simulink model "HVDCVSCBased"  (R2024b)
settings: Solver=ode45  StartTime=0.0  StopTime=3  FixedStep=Ts_Power  RelTol=1e-3  AbsTol=1e-2
InitFcn:
  | Fnom = 50;        % Hz
  | 
  | Fc = 27*Fnom;   % (Hz)
  | Ts_Power = 1/(Fc*100);
  | Ts_Control = Ts_Power*10;
undefined symbols (not defined in the file or in its folder): D1, Delta, DiscIntNeverNeededParam, magnitude
libraries: spsSecondOrderFilterLib x20, spsSeriesRLCBranchLib x14, spsMeanVariableFrequencyLib x12, spsabctoAlphaBetaZeroLib x8, spsThreePhaseVIMeasurementLib x6, spsAlphaBetaZerotodq0Lib x6, spsCurrentMeasurementLib x4, spsThreePhaseHarmonicFilterLib x4, spsVoltageMeasurementLib x4, spsFirstOrderFilterLib x4, spsGroundLib x3, spsThreePhaseSeriesRLCBranchLib x3
(part 2 of 5)

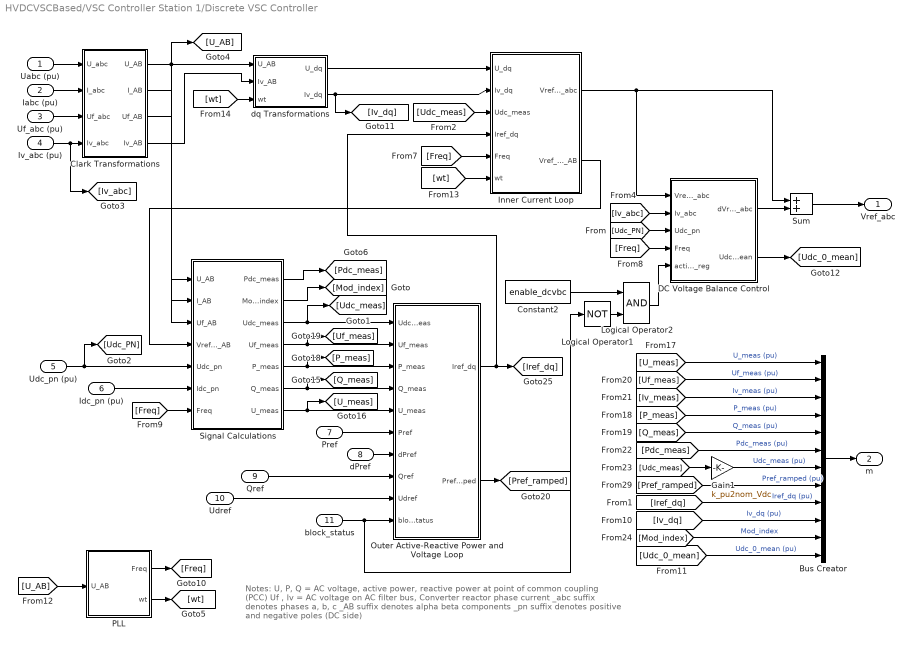
== system HVDCVSCBased/VSC Controller Station 1/Discrete VSC Controller  ==
  note: Notes:
      | U, P, Q = AC voltage, active power, reactive power at point of common coupling (PCC)
      | Uf , Iv  = AC voltage on AC filter bus, Converter reactor phase current
      | _abc suffix denotes phases a, b, c
      | _AB  suffix denotes alpha beta components
      | _pn  suffix denotes positive and negative poles (DC side)
  Uabc (pu) : Inport
  Iabc (pu) : Inport  Port=2
  Uf_abc (pu) : Inport  Port=3
  Iv_abc (pu) : Inport  Port=4
  Udc_pn (pu) : Inport  Port=5
  Idc_pn (pu) : Inport  Port=6
  Pref : Inport  Port=7
  dPref : Inport  Port=8
  Qref : Inport  Port=9
  Udref : Inport  Port=10
  block_status : Inport  Port=11
  Bus Creator : BusCreator  Inputs=12
  Clark Transformations : Subsystem
  Constant2 : Constant  Value=enable_dcvbc
  DC Voltage Balance Control : Subsystem
  Gain1 : Gain  Gain=k_pu2nom_Vdc  SaturateOnIntegerOverflow=on  OutDataTypeStr=Inherit: Same as input  ParamDataTypeStr=Inherit: Same as input
  Inner Current Loop : Subsystem
  Logical Operator1 : Logic  Operator=NOT  Inputs=1  AllPortsSameDT=off
  Logical Operator2 : Logic  AllPortsSameDT=off
  Outer Active-Reactive Power and Voltage Loop : Subsystem
  PLL : Subsystem  mask(Discrete 3-phase PLL){Fmin=f_min_pll, Par_Init=[0   Fnom], ParK=[Kp_pll  Ki_pll], Ts=Ts_Control}
      mask prompts: Fmin "Minimum frequency (Hz):"; Par_Init "Initial inputs:[ Phase(degrees)   Frequency(Hz) ]"; ParK "Regulator gains [ Kp  Ki ]"; Ts "Sample time:"
      mask help:
      | This Phase Locked Loop (PLL) system can be used  to synchronize on a set of variable frequency, three-phase sinusoidal signals.
      |
      | Input 1: Vector containing the normalized
      |              three-phase signals [Va Vb Vc]
      | Output 1:  Measured frequency (Hz) = w/(2pi)
      | Output 2:  Ramp w.t   varying between  0 and 2*pi,
      | synchronized on zero crossings of the fundamental (positive-sequence) of phase A.
      | Output 3: Vector [sin(wt) cos(wt)]
      mask init:
      | Kp=ParK(1);
      | Ki=ParK(2);
      | Phase_Init=Par_Init(1);
      | Finit=Par_Init(2);
  Signal Calculations : Subsystem
  Sum : Sum  SaturateOnIntegerOverflow=on
  dq Transformations : Subsystem
  Vref_abc : Outport  VectorParamsAs1DForOutWhenUnconnected=off
  m : Outport  Port=2  VectorParamsAs1DForOutWhenUnconnected=off
  wires:
  PLL/2(wt) -> [wt]
  PLL/1(Freq) -> [Freq]
  Outer Active-Reactive Power and Voltage Loop/1(Iref_dq) -> Inner Current Loop/4(Iref_dq), [Iref_dq]
  dq Transformations/2(Iv_dq) -> [Iv_dq], Inner Current Loop/2(Iv_dq)
  Inner Current Loop/1(Vref_lim_abc) -> Sum/1, DC Voltage Balance Control/1(Vref_lim_abc)
  dq Transformations/1(U_dq) -> Inner Current Loop/1(U_dq)
  Signal Calculations/3(Udc_meas) -> Outer Active-Reactive Power and Voltage Loop/1(Udc_meas), [Udc_meas]
  Signal Calculations/4(Uf_meas) -> Outer Active-Reactive Power and Voltage Loop/2(Uf_meas), [Uf_meas]
  Signal Calculations/6(Q_meas) -> Outer Active-Reactive Power and Voltage Loop/4(Q_meas), [Q_meas]
  Signal Calculations/5(P_meas) -> Outer Active-Reactive Power and Voltage Loop/3(P_meas), [P_meas]
  Clark Transformations/1(U_AB) -> dq Transformations/1(U_AB), Signal Calculations/1(U_AB), [U_AB]
  Signal Calculations/1(Pdc_meas) -> [Pdc_meas]
  Constant2/1 -> Logical Operator2/1
  Pref/1 -> Outer Active-Reactive Power and Voltage Loop/6(Pref)
  dPref/1 -> Outer Active-Reactive Power and Voltage Loop/7(dPref)
  Qref/1 -> Outer Active-Reactive Power and Voltage Loop/8(Qref)
  Logical Operator2/1 -> DC Voltage Balance Control/5(activate_reg)
  [Udc_PN] -> DC Voltage Balance Control/3(Udc_pn)
  Udc_pn (pu)/1 -> Signal Calculations/5(Udc_pn), [Udc_PN]
  [Iv_abc] -> DC Voltage Balance Control/2(Iv_abc)
  Idc_pn (pu)/1 -> Signal Calculations/6(Idc_pn)
  [Freq] -> Inner Current Loop/5(Freq)
  [Freq] -> DC Voltage Balance Control/4(Freq)
  [Freq] -> Signal Calculations/7(Freq)
  Clark Transformations/2(I_AB) -> Signal Calculations/2(I_AB)
  [U_AB] -> PLL/1(U_AB)
  [wt] -> Inner Current Loop/6(wt)
  [wt] -> dq Transformations/3(wt)
  block_status/1 -> Outer Active-Reactive Power and Voltage Loop/10(block_status), Logical Operator1/1
  Signal Calculations/7(U_meas) -> Outer Active-Reactive Power and Voltage Loop/5(U_meas), [U_meas]
  Sum/1 -> Vref_abc/1
  Logical Operator1/1 -> Logical Operator2/2
  [Udc_meas] -> Inner Current Loop/3(Udc_meas)
  Signal Calculations/2(Mod_index) -> [Mod_index]
  DC Voltage Balance Control/1(dVref_abc) -> Sum/2
  Clark Transformations/4(Iv_AB) -> dq Transformations/2(Iv_AB)
  Clark Transformations/3(Uf_AB) -> Signal Calculations/3(Uf_AB)
  Udref/1 -> Outer Active-Reactive Power and Voltage Loop/9(Udref)
  Bus Creator/1 -> m/1
  [U_meas] -> Bus Creator/1  "U_meas (pu)"
  [P_meas] -> Bus Creator/4  "P_meas (pu)"
  [Uf_meas] -> Bus Creator/2  "Uf_meas (pu)"
  [Iv_meas] -> Bus Creator/3  "Iv_meas (pu)"
  Outer Active-Reactive Power and Voltage Loop/2(Pref_ramped) -> [Pref_ramped]
  [Pref_ramped] -> Bus Creator/8  "Pref_ramped (pu)"
  Inner Current Loop/2(Vref_lim_AB) -> Signal Calculations/4(Vref_lim_AB)
  [Iv_dq] -> Bus Creator/10  "Iv_dq (pu)"
  DC Voltage Balance Control/2(Udc_0_mean) -> [Udc_0_mean]
  [Udc_0_mean] -> Bus Creator/12  "Udc_0_mean (pu)"
  Uabc (pu)/1 -> Clark Transformations/1("U_abc ")
  Iabc (pu)/1 -> Clark Transformations/2("I_abc ")
  Uf_abc (pu)/1 -> Clark Transformations/3("Uf_abc ")
  Iv_abc (pu)/1 -> Clark Transformations/4("Iv_abc "), [Iv_abc]
  [Q_meas] -> Bus Creator/5  "Q_meas (pu)"
  [Pdc_meas] -> Bus Creator/6  "Pdc_meas (pu)"
  [Iref_dq] -> Bus Creator/9  "Iref_dq (pu)"
  [Mod_index] -> Bus Creator/11  "Mod_index"
  Gain1/1 -> Bus Creator/7  "Udc_meas (pu)"
  [Udc_meas] -> Gain1/1

== system HVDCVSCBased/VSC Controller Station 2/Anti-aliasing Filters ==
  note: Filtering
  note: Low-pass filter
  "Uabc " : Inport  PortDimensions=3
  "Iabc " : Inport  Port=2  PortDimensions=3
  "Uf_abc  " : Inport  Port=3  PortDimensions=3
  "Iv_abc " : Inport  Port=4  PortDimensions=3
  "Udc_pn  " : Inport  Port=5
  "Idc_pn " : Inport  Port=6
  Second-Order Filter{,1..5} (6 alike) : spsSecondOrderFilterLib/Second-Order Filter  FilterType=Lowpass  Fo=f0_aa  Zeta=zeta  Ts=Ts_Control  Initialize=off  Vac_Init="[0,  0,  60]"  Vdc_Init=0  PlotResponse=off  FreqRange=[0, 500, 1]
      settings: AttributesFormatString=f0=%<Fo>
  Uabc : Outport  VectorParamsAs1DForOutWhenUnconnected=off
  Iabc : Outport  Port=2  VectorParamsAs1DForOutWhenUnconnected=off
  Uf_abc : Outport  Port=3  VectorParamsAs1DForOutWhenUnconnected=off
  " Iv_abc" : Outport  Port=4  VectorParamsAs1DForOutWhenUnconnected=off
  "Udc_pn " : Outport  Port=5  VectorParamsAs1DForOutWhenUnconnected=off
  " Idc_pn" : Outport  Port=6  VectorParamsAs1DForOutWhenUnconnected=off
  wires:
  "Iv_abc "/1 -> Second-Order Filter/1
  Second-Order Filter/1 -> " Iv_abc"/1
  "Uf_abc  "/1 -> Second-Order Filter1/1
  Second-Order Filter1/1 -> Uf_abc/1
  "Uabc "/1 -> Second-Order Filter2/1
  Second-Order Filter2/1 -> Uabc/1
  "Udc_pn  "/1 -> Second-Order Filter3/1
  Second-Order Filter3/1 -> "Udc_pn "/1
  "Idc_pn "/1 -> Second-Order Filter4/1
  Second-Order Filter4/1 -> " Idc_pn"/1
  "Iabc "/1 -> Second-Order Filter5/1
  Second-Order Filter5/1 -> Iabc/1

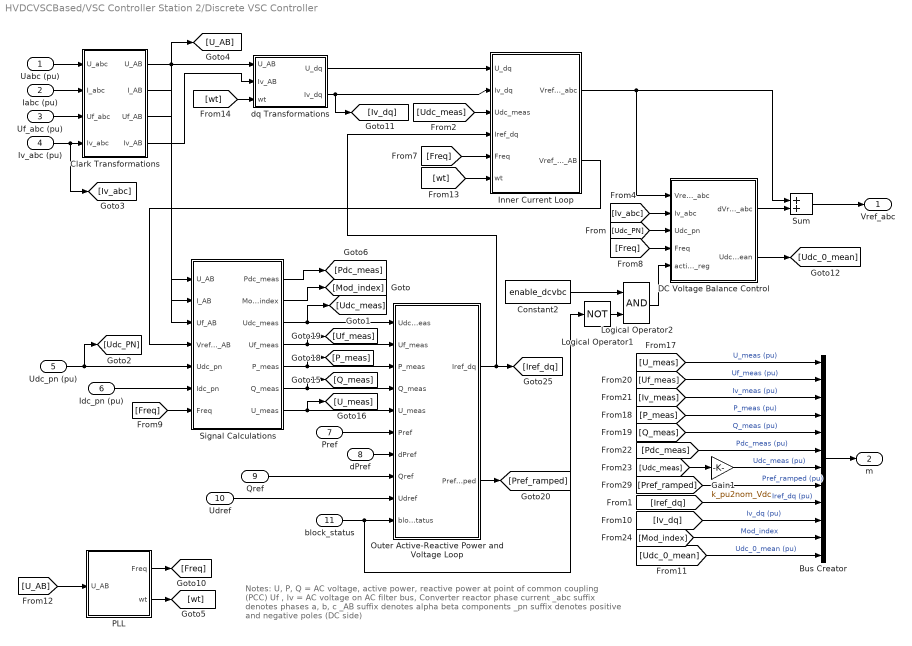
== system HVDCVSCBased/VSC Controller Station 2/Discrete VSC Controller  ==
  note: Notes:
      | U, P, Q = AC voltage, active power, reactive power at point of common coupling (PCC)
      | Uf , Iv  = AC voltage on AC filter bus, Converter reactor phase current
      | _abc suffix denotes phases a, b, c
      | _AB  suffix denotes alpha beta components
      | _pn  suffix denotes positive and negative poles (DC side)
  Uabc (pu) : Inport
  Iabc (pu) : Inport  Port=2
  Uf_abc (pu) : Inport  Port=3
  Iv_abc (pu) : Inport  Port=4
  Udc_pn (pu) : Inport  Port=5
  Idc_pn (pu) : Inport  Port=6
  Pref : Inport  Port=7
  dPref : Inport  Port=8
  Qref : Inport  Port=9
  Udref : Inport  Port=10
  block_status : Inport  Port=11
  Bus Creator : BusCreator  Inputs=12
  Clark Transformations : Subsystem
  Constant2 : Constant  Value=enable_dcvbc
  DC Voltage Balance Control : Subsystem
  Gain1 : Gain  Gain=k_pu2nom_Vdc  SaturateOnIntegerOverflow=on  OutDataTypeStr=Inherit: Same as input  ParamDataTypeStr=Inherit: Same as input
  Inner Current Loop : Subsystem
  Logical Operator1 : Logic  Operator=NOT  Inputs=1  AllPortsSameDT=off
  Logical Operator2 : Logic  AllPortsSameDT=off
  Outer Active-Reactive Power and Voltage Loop : Subsystem
  PLL : Subsystem  mask(Discrete 3-phase PLL){Fmin=f_min_pll, Par_Init=[0   Fnom], ParK=[Kp_pll  Ki_pll], Ts=Ts_Control}
      mask prompts: Fmin "Minimum frequency (Hz):"; Par_Init "Initial inputs:[ Phase(degrees)   Frequency(Hz) ]"; ParK "Regulator gains [ Kp  Ki ]"; Ts "Sample time:"
      mask help:
      | This Phase Locked Loop (PLL) system can be used  to synchronize on a set of variable frequency, three-phase sinusoidal signals.
      |
      | Input 1: Vector containing the normalized
      |              three-phase signals [Va Vb Vc]
      | Output 1:  Measured frequency (Hz) = w/(2pi)
      | Output 2:  Ramp w.t   varying between  0 and 2*pi,
      | synchronized on zero crossings of the fundamental (positive-sequence) of phase A.
      | Output 3: Vector [sin(wt) cos(wt)]
      mask init:
      | Kp=ParK(1);
      | Ki=ParK(2);
      | Phase_Init=Par_Init(1);
      | Finit=Par_Init(2);
  Signal Calculations : Subsystem
  Sum : Sum  SaturateOnIntegerOverflow=on
  dq Transformations : Subsystem
  Vref_abc : Outport  VectorParamsAs1DForOutWhenUnconnected=off
  m : Outport  Port=2  VectorParamsAs1DForOutWhenUnconnected=off
  wires:
  PLL/2(wt) -> [wt]
  PLL/1(Freq) -> [Freq]
  Outer Active-Reactive Power and Voltage Loop/1(Iref_dq) -> Inner Current Loop/4(Iref_dq), [Iref_dq]
  dq Transformations/2(Iv_dq) -> [Iv_dq], Inner Current Loop/2(Iv_dq)
  Inner Current Loop/1(Vref_lim_abc) -> Sum/1, DC Voltage Balance Control/1(Vref_lim_abc)
  dq Transformations/1(U_dq) -> Inner Current Loop/1(U_dq)
  Signal Calculations/3(Udc_meas) -> Outer Active-Reactive Power and Voltage Loop/1(Udc_meas), [Udc_meas]
  Signal Calculations/4(Uf_meas) -> Outer Active-Reactive Power and Voltage Loop/2(Uf_meas), [Uf_meas]
  Signal Calculations/6(Q_meas) -> Outer Active-Reactive Power and Voltage Loop/4(Q_meas), [Q_meas]
  Signal Calculations/5(P_meas) -> Outer Active-Reactive Power and Voltage Loop/3(P_meas), [P_meas]
  Clark Transformations/1(U_AB) -> dq Transformations/1(U_AB), Signal Calculations/1(U_AB), [U_AB]
  Signal Calculations/1(Pdc_meas) -> [Pdc_meas]
  Constant2/1 -> Logical Operator2/1
  Pref/1 -> Outer Active-Reactive Power and Voltage Loop/6(Pref)
  dPref/1 -> Outer Active-Reactive Power and Voltage Loop/7(dPref)
  Qref/1 -> Outer Active-Reactive Power and Voltage Loop/8(Qref)
  Logical Operator2/1 -> DC Voltage Balance Control/5(activate_reg)
  [Udc_PN] -> DC Voltage Balance Control/3(Udc_pn)
  Udc_pn (pu)/1 -> Signal Calculations/5(Udc_pn), [Udc_PN]
  [Iv_abc] -> DC Voltage Balance Control/2(Iv_abc)
  Idc_pn (pu)/1 -> Signal Calculations/6(Idc_pn)
  [Freq] -> Inner Current Loop/5(Freq)
  [Freq] -> DC Voltage Balance Control/4(Freq)
  [Freq] -> Signal Calculations/7(Freq)
  Clark Transformations/2(I_AB) -> Signal Calculations/2(I_AB)
  [U_AB] -> PLL/1(U_AB)
  [wt] -> Inner Current Loop/6(wt)
  [wt] -> dq Transformations/3(wt)
  block_status/1 -> Outer Active-Reactive Power and Voltage Loop/10(block_status), Logical Operator1/1
  Signal Calculations/7(U_meas) -> Outer Active-Reactive Power and Voltage Loop/5(U_meas), [U_meas]
  Sum/1 -> Vref_abc/1
  Logical Operator1/1 -> Logical Operator2/2
  [Udc_meas] -> Inner Current Loop/3(Udc_meas)
  Signal Calculations/2(Mod_index) -> [Mod_index]
  DC Voltage Balance Control/1(dVref_abc) -> Sum/2
  Clark Transformations/4(Iv_AB) -> dq Transformations/2(Iv_AB)
  Clark Transformations/3(Uf_AB) -> Signal Calculations/3(Uf_AB)
  Udref/1 -> Outer Active-Reactive Power and Voltage Loop/9(Udref)
  Bus Creator/1 -> m/1
  [U_meas] -> Bus Creator/1  "U_meas (pu)"
  [P_meas] -> Bus Creator/4  "P_meas (pu)"
  [Uf_meas] -> Bus Creator/2  "Uf_meas (pu)"
  [Iv_meas] -> Bus Creator/3  "Iv_meas (pu)"
  Outer Active-Reactive Power and Voltage Loop/2(Pref_ramped) -> [Pref_ramped]
  [Pref_ramped] -> Bus Creator/8  "Pref_ramped (pu)"
  Inner Current Loop/2(Vref_lim_AB) -> Signal Calculations/4(Vref_lim_AB)
  [Iv_dq] -> Bus Creator/10  "Iv_dq (pu)"
  DC Voltage Balance Control/2(Udc_0_mean) -> [Udc_0_mean]
  [Udc_0_mean] -> Bus Creator/12  "Udc_0_mean (pu)"
  Uabc (pu)/1 -> Clark Transformations/1("U_abc ")
  Iabc (pu)/1 -> Clark Transformations/2("I_abc ")
  Uf_abc (pu)/1 -> Clark Transformations/3("Uf_abc ")
  Iv_abc (pu)/1 -> Clark Transformations/4("Iv_abc "), [Iv_abc]
  [Q_meas] -> Bus Creator/5  "Q_meas (pu)"
  [Pdc_meas] -> Bus Creator/6  "Pdc_meas (pu)"
  [Iref_dq] -> Bus Creator/9  "Iref_dq (pu)"
  [Mod_index] -> Bus Creator/11  "Mod_index"
  Gain1/1 -> Bus Creator/7  "Udc_meas (pu)"
  [Udc_meas] -> Gain1/1

== system HVDCVSCBased/VSC Controller Station 1/Discrete VSC Controller /Clark Transformations ==
  note: 0: Y-Y
      | 1: Y-D1
      | 2: Y-D11
  note: Clark's Transformations
  "U_abc " : Inport
  "I_abc " : Inport  Port=2
  "Uf_abc " : Inport  Port=3
  "Iv_abc " : Inport  Port=4
  CLARK  with Rotating reference : Subsystem
  CLARK  with Rotating reference1 : Subsystem
  Constant2 : Constant  Value=Tr_connection
  Selector{,1..3} (4 alike) : Selector  InputPortWidth=3  IndexOptions=Index vector (dialog)  Indices=[1 2]  OutputSizes=1
  abc to Alpha-Beta-Zero : spsabctoAlphaBetaZeroLib/abc to Alpha-Beta-Zero
  abc to Alpha-Beta-Zero1 : spsabctoAlphaBetaZeroLib/abc to Alpha-Beta-Zero
  U_AB : Outport  VectorParamsAs1DForOutWhenUnconnected=off
  I_AB : Outport  Port=2  VectorParamsAs1DForOutWhenUnconnected=off
  Uf_AB : Outport  Port=3  VectorParamsAs1DForOutWhenUnconnected=off
  Iv_AB : Outport  Port=4  VectorParamsAs1DForOutWhenUnconnected=off
  wires:
  Constant2/1 -> CLARK  with Rotating reference/2(Type), CLARK  with Rotating reference1/2(Type)
  "U_abc "/1 -> CLARK  with Rotating reference/1(abc)
  "I_abc "/1 -> CLARK  with Rotating reference1/1(abc)
  "Uf_abc "/1 -> abc to Alpha-Beta-Zero/1
  "Iv_abc "/1 -> abc to Alpha-Beta-Zero1/1
  CLARK  with Rotating reference/1(AB0) -> Selector/1
  abc to Alpha-Beta-Zero/1 -> Selector2/1
  abc to Alpha-Beta-Zero1/1 -> Selector3/1
  CLARK  with Rotating reference1/1(AB0) -> Selector1/1
  Selector/1 -> U_AB/1
  Selector1/1 -> I_AB/1
  Selector2/1 -> Uf_AB/1
  Selector3/1 -> Iv_AB/1

== system HVDCVSCBased/VSC Controller Station 1/Discrete VSC Controller /DC Voltage Balance Control ==
  note: DC Voltage Balance Control
  note: pu AC ==> pu DC
  Vref_lim_abc : Inport
  Iv_abc : Inport  Port=2
  Udc_pn : Inport  Port=3
  Freq : Inport  Port=4
  activate_reg : Inport  Port=5
  Constant8 : Constant  Value=0
  First-Order Filter : spsFirstOrderFilterLib/First-Order Filter  FilterType=Lowpass  Tc=1/(2*pi*f0_dcvbc)  Ts=Ts_Control  Initialize=off  Vac_Init=[0, 0, 60]  Vdc_Init=0  PlotResponse=off  FreqRange="[0,  200,  1]"
      settings: AttributesFormatString=Tc:%<Tc>
  Gain4 : Gain  Gain=k_pu2nom_Vdc  SaturateOnIntegerOverflow=on  OutDataTypeStr=Inherit: Same as input  ParamDataTypeStr=Inherit: Same as input
  Mean (Variable Frequency) : spsMeanVariableFrequencyLib/Mean (Variable Frequency)  Finit=Fnom  Fmin=f_min_pll  Vinit=0  Ts=Ts_Control
  Regulator : Subsystem  TreatAsAtomicUnit=on
  Sum : Sum  Inputs=1  SaturateOnIntegerOverflow=on
  Switch2 : Switch  Criteria=u2 > Threshold  InputSameDT=off
  dVref_abc : Outport  VectorParamsAs1DForOutWhenUnconnected=off
  Udc_0_mean : Outport  Port=2  VectorParamsAs1DForOutWhenUnconnected=off
  wires:
  First-Order Filter/1 -> Mean (Variable Frequency)/2
  Sum/1 -> First-Order Filter/1
  Freq/1 -> Mean (Variable Frequency)/1
  Vref_lim_abc/1 -> Regulator/1(V_ref_lim_abc)
  Iv_abc/1 -> Regulator/2(Iv_abc)
  Udc_pn/1 -> Sum/1
  Mean (Variable Frequency)/1 -> Gain4/1
  Gain4/1 -> Regulator/3(Udc_0_mean), Udc_0_mean/1
  Regulator/1(dV_ref_abc_dcvbc) -> Switch2/1
  Switch2/1 -> dVref_abc/1
  Constant8/1 -> Switch2/3
  activate_reg/1 -> Regulator/Enable, Switch2/2

== system HVDCVSCBased/VSC Controller Station 1/Discrete VSC Controller /Inner Current Loop ==
  note: Inner Current Loop
  U_dq : Inport
  Iv_dq : Inport  Port=2
  Udc_meas : Inport  Port=3
  Iref_dq : Inport  Port=4
  Freq : Inport  Port=5
  wt : Inport  Port=6
  AC_Current_Control : Subsystem
  Alpha-Beta-Zero to abc : spsAlphaBetaZerotoabcLib/Alpha-Beta-Zero to abc
  Constant1 : Constant  Value=0
  Max=10 Min=0 : Saturate  UpperLimit=10  LowerLimit=0
  Mean (Variable Frequency IC = 1.0 ) : spsMeanVariableFrequencyLib/Mean (Variable Frequency)  Finit=Fnom  Fmin=f_min_pll  Vinit=1.0  Ts=Ts_Control
  Mux1 : Mux  Inputs=[2 1]
  Reference_Voltage_Conditioning : Subsystem
  Reference_Voltage_Limitation : Subsystem
  Selector : Selector  InputPortWidth=3  IndexOptions=Index vector (dialog)  Indices=[ 1 2]  OutputSizes=1
  dq0 to Alpha-Beta-Zero : spsdq0toAlphaBetaZeroLib/dq0 to Alpha-Beta-Zero  Alignment=90 degrees behind phase A axis
  Vref_lim_abc : Outport  VectorParamsAs1DForOutWhenUnconnected=off
  Vref_lim_AB : Outport  Port=2  VectorParamsAs1DForOutWhenUnconnected=off
  wires:
  Udc_meas/1 -> Mean (Variable Frequency IC = 1.0 )/2
  Selector/1 -> Vref_lim_AB/1
  Reference_Voltage_Limitation/1(Vref_lim_dq) -> Mux1/1
  Alpha-Beta-Zero to abc/1 -> Vref_lim_abc/1
  Mux1/1 -> dq0 to Alpha-Beta-Zero/1
  Constant1/1 -> Mux1/2
  wt/1 -> dq0 to Alpha-Beta-Zero/2
  dq0 to Alpha-Beta-Zero/1 -> Selector/1, Alpha-Beta-Zero to abc/1
  Mean (Variable Frequency IC = 1.0 )/1 -> Max=10 Min=0/1
  Freq/1 -> Mean (Variable Frequency IC = 1.0 )/1, AC_Current_Control/4(Freq)
  Iref_dq/1 -> AC_Current_Control/2(Iref_dq)
  U_dq/1 -> AC_Current_Control/3(U_dq)
  Reference_Voltage_Conditioning/1(Vref_dq) -> Reference_Voltage_Limitation/1(Vref_dq)
  AC_Current_Control/1(Vref_dq_tmp) -> Reference_Voltage_Conditioning/1(Vref_dq_tmp)
  Max=10 Min=0/1 -> Reference_Voltage_Conditioning/2(Udc_meas_mean)
  Iv_dq/1 -> AC_Current_Control/1(Iv_dq)

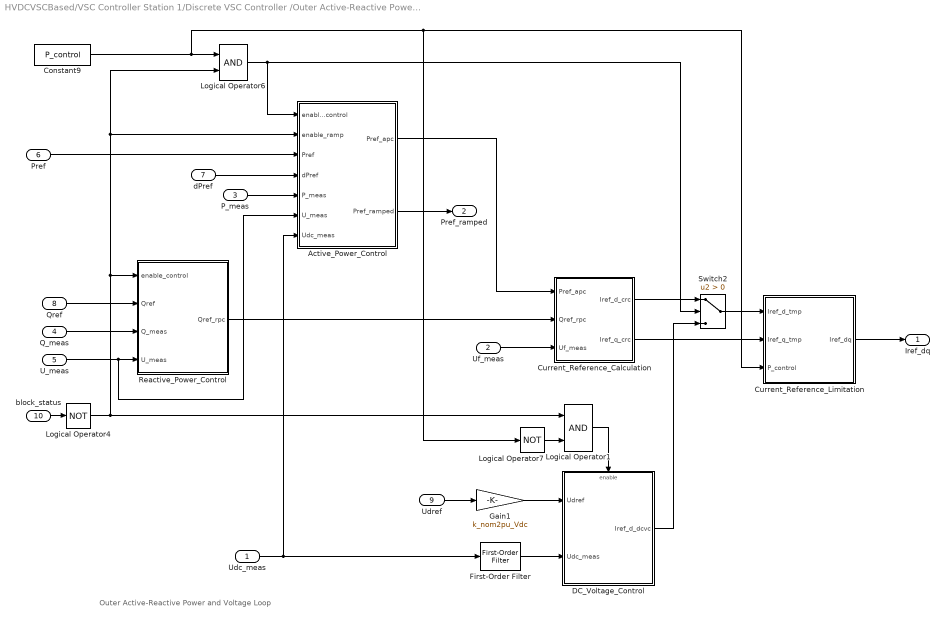
== system HVDCVSCBased/VSC Controller Station 1/Discrete VSC Controller /Outer Active-Reactive Power and Voltage Loop ==
  note: Outer Active-Reactive Power and Voltage Loop
  Udc_meas : Inport
  Uf_meas : Inport  Port=2
  P_meas : Inport  Port=3
  Q_meas : Inport  Port=4
  U_meas : Inport  Port=5
  Pref : Inport  Port=6
  dPref : Inport  Port=7
  Qref : Inport  Port=8
  Udref : Inport  Port=9
  block_status : Inport  Port=10
  Active_Power_Control : Subsystem
  Constant9 : Constant  Value=P_control
  Current_Reference_Calculation : Subsystem
  Current_Reference_Limitation : Subsystem
  DC_Voltage_Control : Subsystem
  First-Order Filter : spsFirstOrderFilterLib/First-Order Filter  FilterType=Lowpass  Tc=1/(2*pi*f0_Udc)  Ts=Ts_Control  Initialize=on  Vac_Init=[0, 0, 60]  Vdc_Init=k_nom2pu_Vdc  PlotResponse=off  FreqRange="[0,  200,  1]"
      settings: AttributesFormatString=Tc:%<Tc>\nIC:%<Vdc_Init>
  Gain1 : Gain  Gain=k_nom2pu_Vdc  SaturateOnIntegerOverflow=on  OutDataTypeStr=Inherit: Same as input  ParamDataTypeStr=Inherit: Same as input
      settings: AttributesFormatString=Gain:%<Gain>
  Logical Operator1 : Logic  AllPortsSameDT=off
  Logical Operator4 : Logic  Operator=NOT  AllPortsSameDT=off
  Logical Operator6 : Logic  AllPortsSameDT=off
  Logical Operator7 : Logic  Operator=NOT  AllPortsSameDT=off
  Reactive_Power_Control : Subsystem
  Switch2 : Switch  Criteria=u2 > Threshold  InputSameDT=off
  Iref_dq : Outport  VectorParamsAs1DForOutWhenUnconnected=off
  Pref_ramped : Outport  Port=2  VectorParamsAs1DForOutWhenUnconnected=off
  wires:
  First-Order Filter/1 -> DC_Voltage_Control/2(Udc_meas)
  Udref/1 -> Gain1/1
  Gain1/1 -> DC_Voltage_Control/1(Udref)
  Logical Operator1/1 -> DC_Voltage_Control/Enable
  Current_Reference_Limitation/1(Iref_dq) -> Iref_dq/1
  Switch2/1 -> Current_Reference_Limitation/1(Iref_d_tmp)
  Logical Operator4/1 -> Logical Operator1/1, Logical Operator6/2, Active_Power_Control/2(enable_ramp), Reactive_Power_Control/1(enable_control)
  Current_Reference_Calculation/1(Iref_d_crc) -> Switch2/1
  Q_meas/1 -> Reactive_Power_Control/3(Q_meas)
  P_meas/1 -> Active_Power_Control/5(P_meas)
  DC_Voltage_Control/1(Iref_d_dcvc) -> Switch2/3
  Udc_meas/1 -> Active_Power_Control/7(Udc_meas), First-Order Filter/1
  block_status/1 -> Logical Operator4/1
  Constant9/1 -> Logical Operator6/1, Current_Reference_Limitation/3(P_control), Logical Operator7/1
  Logical Operator6/1 -> Switch2/2, Active_Power_Control/1(enable_control)
  U_meas/1 -> Reactive_Power_Control/4(U_meas), Active_Power_Control/6(U_meas)
  Current_Reference_Calculation/2(Iref_q_crc) -> Current_Reference_Limitation/2(Iref_q_tmp)
  dPref/1 -> Active_Power_Control/4(dPref)
  Active_Power_Control/1(Pref_apc) -> Current_Reference_Calculation/1(Pref_apc)
  Reactive_Power_Control/1(Qref_rpc) -> Current_Reference_Calculation/2(Qref_rpc)
  Pref/1 -> Active_Power_Control/3(Pref)
  Uf_meas/1 -> Current_Reference_Calculation/3(Uf_meas)
  Qref/1 -> Reactive_Power_Control/2(Qref)
  Logical Operator7/1 -> Logical Operator1/2
  Active_Power_Control/2(Pref_ramped) -> Pref_ramped/1

== system HVDCVSCBased/VSC Controller Station 1/Discrete VSC Controller /PLL ==
  note: Discrete 3-phase PLL (Variation)
  U_AB : Inport
  Alpha-Beta-Zero to dq0 : spsAlphaBetaZerotodq0Lib/Alpha-Beta-Zero to dq0  Alignment=90 degrees behind phase A axis
  Constant1 : Constant  Value=0
  Constant4 : Constant  Value=2*pi
  Discrete PI Controller : Subsystem  DialogController=POWERSYS.PowerSysDialog  mask(Discrete PI Controller){Kp=Kp, Ki=Ki, Par_Limits=2*pi*Finit*[1.25 0.75], Init=2*pi*Finit, Ts=Ts}
      mask prompts: Kp "Proportional gain (Kp):"; Ki "Integral gain (Ki):"; Par_Limits "Output limits: [ Upper   Lower ]"; Init "Output initial value:"; Ts "Sample time:"
      mask help: This block implements a discrete PI controller.
      mask init:
      | UpperLimit=Par_Limits(1);
      | LowerLimit=Par_Limits(2);
      | power_initmask();
      mask Help: This block is part of a subset of blocks in the Extras library that does not have documentation associated with it, other than the block mask description.
      mask Display: disp('PI');
  Discrete Rate Limiter : Subsystem  DialogController=POWERSYS.PowerSysDialog  mask(Discrete Rate Limiter){R=12, F=-12, Vinit=Finit, Ts=Ts}
      mask prompts: R "Rising slew rate:"; F "Falling slew rate:"; Vinit "Initial input:"; Ts "Sample time:"
      mask help: DISCRETE BLOCK : Limit rising and falling rates of signal
      mask init:
      | UpperLimit=R*Ts;
      | LowerLimit=F*Ts;
      | power_initmask();
      mask Help: This block is part of a subset of blocks in the Extras library that does not have documentation associated with it, other than the block mask description.
      mask Display: disp('Discrete\nRate\nLimiter')
  Discrete-Time Integrator : DiscreteIntegrator  InitialCondition=Phase_Init*pi/180  SampleTime=Ts  ICPrevOutput=DiscIntNeverNeededParam  ICPrevScaledInput=DiscIntNeverNeededParam
  Gain10 : Gain  Gain=1/2/pi  SaturateOnIntegerOverflow=on  OutDataTypeStr=Inherit: Same as input  ParamDataTypeStr=Inherit: Same as input
  Math Function : Math  Operator=mod  SignedPower=on
  Mean (Variable Frequency) : spsMeanVariableFrequencyLib/Mean (Variable Frequency)  Finit=Finit  Fmin=Fmin  Vinit=0  Ts=Ts
  Mux1 : Mux  Inputs=[2 1]
  Second-Order Filter : spsSecondOrderFilterLib/Second-Order Filter  FilterType=Lowpass  Fo=25  Zeta=0.707  Ts=Ts  Initialize=on  Vac_Init=[0 0 Finit]  Vdc_Init=Finit  PlotResponse=off  FreqRange=[0, 500, 1]
  Selector : Selector  InputPortWidth=3  IndexOptions=Index vector (dialog)  Indices=2  OutputSizes=1
  Unit Delay : UnitDelay  InitialCondition=Finit  SampleTime=Ts  HasFrameUpgradeWarning=on
  Freq : Outport  VectorParamsAs1DForOutWhenUnconnected=off
  wt : Outport  Port=2  VectorParamsAs1DForOutWhenUnconnected=off
  wires:
  Constant1/1 -> Mux1/2
  Mux1/1 -> Alpha-Beta-Zero to dq0/1
  U_AB/1 -> Mux1/1
  Mean (Variable Frequency)/1 -> Discrete PI Controller/1(Error)
  Alpha-Beta-Zero to dq0/1 -> Selector/1
  Constant4/1 -> Math Function/2
  Discrete-Time Integrator/1 -> Math Function/1
  Math Function/1 -> wt/1, Alpha-Beta-Zero to dq0/2
  Discrete PI Controller/1(Out) -> Discrete-Time Integrator/1, Gain10/1  "W"
  Gain10/1 -> Discrete Rate Limiter/1(In)
  Discrete Rate Limiter/1(Out) -> Second-Order Filter/1
  Unit Delay/1 -> Freq/1, Mean (Variable Frequency)/1
  Second-Order Filter/1 -> Unit Delay/1
  Selector/1 -> Mean (Variable Frequency)/2  "Vq"

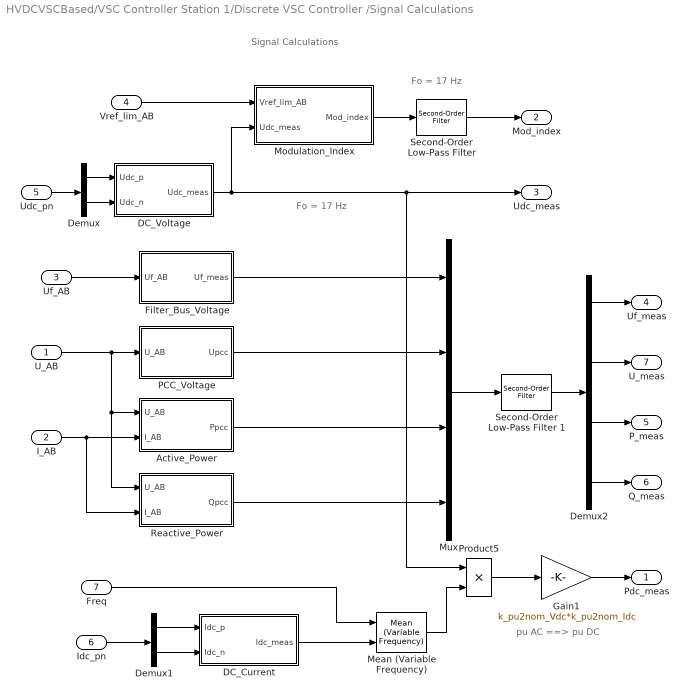
== system HVDCVSCBased/VSC Controller Station 1/Discrete VSC Controller /Signal Calculations ==
  note: Fo = 17 Hz
  note: Fo = 17 Hz
  note: Signal Calculations
  note: pu AC ==> pu DC
  U_AB : Inport
  I_AB : Inport  Port=2
  Uf_AB : Inport  Port=3
  Vref_lim_AB : Inport  Port=4
  Udc_pn : Inport  Port=5
  Idc_pn : Inport  Port=6
  Freq : Inport  Port=7
  Active_Power : Subsystem
  DC_Current : Subsystem
  DC_Voltage : Subsystem
  Demux : Demux  Outputs=2
      settings: DisplayOption=none
  Demux1 : Demux  Outputs=2
      settings: DisplayOption=none
  Demux2 : Demux
  Filter_Bus_Voltage : Subsystem
  Gain1 : Gain  Gain=k_pu2nom_Vdc*k_pu2nom_Idc  SaturateOnIntegerOverflow=on  OutDataTypeStr=Inherit: Same as input  ParamDataTypeStr=Inherit: Same as input
  "Mean (Variable Frequency) " : spsMeanVariableFrequencyLib/Mean (Variable Frequency)  Finit=Fnom  Fmin=f_min_pll  Vinit=0  Ts=Ts_Control
  Modulation_Index : Subsystem
  Mux : Mux
  PCC_Voltage : Subsystem
  Product5 : Product  SaturateOnIntegerOverflow=on  OutDataTypeStr=Inherit: Same as first input
  Reactive_Power : Subsystem
  "Second-Order Low-Pass Filter " : spsSecondOrderFilterLib/Second-Order Filter  FilterType=Lowpass  Fo=f0_sc  Zeta=zeta_sc  Ts=Ts_Control  Initialize=off  Vac_Init="[0,  0,  60]"  Vdc_Init=0  PlotResponse=off  FreqRange=[0, 500, 1]
      settings: AttributesFormatString=f0=%<Fo>
  Second-Order Low-Pass Filter 1 : spsSecondOrderFilterLib/Second-Order Filter  FilterType=Lowpass  Fo=f0_sc  Zeta=zeta_sc  Ts=Ts_Control  Initialize=off  Vac_Init="[0,  0,  60]"  Vdc_Init=0  PlotResponse=off  FreqRange=[0, 500, 1]
      settings: AttributesFormatString=f0=%<Fo>
  Pdc_meas : Outport  VectorParamsAs1DForOutWhenUnconnected=off
  Mod_index : Outport  Port=2  VectorParamsAs1DForOutWhenUnconnected=off
  Udc_meas : Outport  Port=3  VectorParamsAs1DForOutWhenUnconnected=off
  Uf_meas : Outport  Port=4  VectorParamsAs1DForOutWhenUnconnected=off
  P_meas : Outport  Port=5  VectorParamsAs1DForOutWhenUnconnected=off
  Q_meas : Outport  Port=6  VectorParamsAs1DForOutWhenUnconnected=off
  U_meas : Outport  Port=7  VectorParamsAs1DForOutWhenUnconnected=off
  wires:
  Demux2/4 -> Q_meas/1
  Demux2/3 -> P_meas/1
  Demux2/2 -> U_meas/1
  Demux2/1 -> Uf_meas/1
  Reactive_Power/1(Qpcc) -> Mux/4
  Active_Power/1(Ppcc) -> Mux/3
  PCC_Voltage/1(Upcc) -> Mux/2
  Filter_Bus_Voltage/1(Uf_meas) -> Mux/1
  "Second-Order Low-Pass Filter "/1 -> Mod_index/1
  Modulation_Index/1(Mod_index) -> "Second-Order Low-Pass Filter "/1
  Second-Order Low-Pass Filter 1/1 -> Demux2/1
  Mux/1 -> Second-Order Low-Pass Filter 1/1
  Gain1/1 -> Pdc_meas/1
  Freq/1 -> "Mean (Variable Frequency) "/1
  Product5/1 -> Gain1/1
  "Mean (Variable Frequency) "/1 -> Product5/2
  Demux/2 -> DC_Voltage/2(Udc_n)
  Uf_AB/1 -> Filter_Bus_Voltage/1(Uf_AB)
  U_AB/1 -> PCC_Voltage/1(U_AB), Active_Power/1(U_AB), Reactive_Power/1(U_AB)
  I_AB/1 -> Active_Power/2(I_AB), Reactive_Power/2(I_AB)
  DC_Voltage/1(Udc_meas) -> Product5/1, Udc_meas/1, Modulation_Index/2(Udc_meas)
  DC_Current/1(Idc_meas) -> "Mean (Variable Frequency) "/2
  Udc_pn/1 -> Demux/1
  Demux/1 -> DC_Voltage/1(Udc_p)
  Demux1/1 -> DC_Current/1(Idc_p)
  Demux1/2 -> DC_Current/2(Idc_n)
  Idc_pn/1 -> Demux1/1
  Vref_lim_AB/1 -> Modulation_Index/1(Vref_lim_AB)

== system HVDCVSCBased/VSC Controller Station 1/Discrete VSC Controller /dq Transformations ==
  note: dq Transformations
  U_AB : Inport
  Iv_AB : Inport  Port=2
  wt : Inport  Port=3
  Alpha-Beta-Zero to dq0 : spsAlphaBetaZerotodq0Lib/Alpha-Beta-Zero to dq0  Alignment=90 degrees behind phase A axis
  "Alpha-Beta-Zero to dq0 " : spsAlphaBetaZerotodq0Lib/Alpha-Beta-Zero to dq0  Alignment=90 degrees behind phase A axis
  Constant1 : Constant  Value=0
  Mux1 : Mux  Inputs=[2 1]
  Mux4 : Mux  Inputs=[2 1]
  Selector : Selector  InputPortWidth=3  IndexOptions=Index vector (dialog)  Indices=[1 2]  OutputSizes=1
  Selector3 : Selector  InputPortWidth=3  IndexOptions=Index vector (dialog)  Indices=[1 2]  OutputSizes=1
  U_dq : Outport  VectorParamsAs1DForOutWhenUnconnected=off
  Iv_dq : Outport  Port=2  VectorParamsAs1DForOutWhenUnconnected=off
  wires:
  wt/1 -> Alpha-Beta-Zero to dq0/2, "Alpha-Beta-Zero to dq0 "/2
  Constant1/1 -> Mux4/2, Mux1/2
  Mux4/1 -> "Alpha-Beta-Zero to dq0 "/1
  Iv_AB/1 -> Mux4/1
  Mux1/1 -> Alpha-Beta-Zero to dq0/1
  U_AB/1 -> Mux1/1
  "Alpha-Beta-Zero to dq0 "/1 -> Selector3/1
  Alpha-Beta-Zero to dq0/1 -> Selector/1
  Selector/1 -> U_dq/1
  Selector3/1 -> Iv_dq/1

== system HVDCVSCBased/VSC Controller Station 2/Discrete VSC Controller /Clark Transformations ==
  note: 0: Y-Y
      | 1: Y-D1
      | 2: Y-D11
  note: Clark's Transformations
  "U_abc " : Inport
  "I_abc " : Inport  Port=2
  "Uf_abc " : Inport  Port=3
  "Iv_abc " : Inport  Port=4
  CLARK  with Rotating reference : Subsystem
  CLARK  with Rotating reference1 : Subsystem
  Constant2 : Constant  Value=Tr_connection
  Selector{,1..3} (4 alike) : Selector  InputPortWidth=3  IndexOptions=Index vector (dialog)  Indices=[1 2]  OutputSizes=1
  abc to Alpha-Beta-Zero : spsabctoAlphaBetaZeroLib/abc to Alpha-Beta-Zero
  abc to Alpha-Beta-Zero1 : spsabctoAlphaBetaZeroLib/abc to Alpha-Beta-Zero
  U_AB : Outport  VectorParamsAs1DForOutWhenUnconnected=off
  I_AB : Outport  Port=2  VectorParamsAs1DForOutWhenUnconnected=off
  Uf_AB : Outport  Port=3  VectorParamsAs1DForOutWhenUnconnected=off
  Iv_AB : Outport  Port=4  VectorParamsAs1DForOutWhenUnconnected=off
  wires:
  Constant2/1 -> CLARK  with Rotating reference/2(Type), CLARK  with Rotating reference1/2(Type)
  "U_abc "/1 -> CLARK  with Rotating reference/1(abc)
  "I_abc "/1 -> CLARK  with Rotating reference1/1(abc)
  "Uf_abc "/1 -> abc to Alpha-Beta-Zero/1
  "Iv_abc "/1 -> abc to Alpha-Beta-Zero1/1
  CLARK  with Rotating reference/1(AB0) -> Selector/1
  abc to Alpha-Beta-Zero/1 -> Selector2/1
  abc to Alpha-Beta-Zero1/1 -> Selector3/1
  CLARK  with Rotating reference1/1(AB0) -> Selector1/1
  Selector/1 -> U_AB/1
  Selector1/1 -> I_AB/1
  Selector2/1 -> Uf_AB/1
  Selector3/1 -> Iv_AB/1

== system HVDCVSCBased/VSC Controller Station 2/Discrete VSC Controller /DC Voltage Balance Control ==
  note: DC Voltage Balance Control
  note: pu AC ==> pu DC
  Vref_lim_abc : Inport
  Iv_abc : Inport  Port=2
  Udc_pn : Inport  Port=3
  Freq : Inport  Port=4
  activate_reg : Inport  Port=5
  Constant8 : Constant  Value=0
  First-Order Filter : spsFirstOrderFilterLib/First-Order Filter  FilterType=Lowpass  Tc=1/(2*pi*f0_dcvbc)  Ts=Ts_Control  Initialize=off  Vac_Init=[0, 0, 60]  Vdc_Init=0  PlotResponse=off  FreqRange="[0,  200,  1]"
      settings: AttributesFormatString=Tc:%<Tc>
  Gain4 : Gain  Gain=k_pu2nom_Vdc  SaturateOnIntegerOverflow=on  OutDataTypeStr=Inherit: Same as input  ParamDataTypeStr=Inherit: Same as input
  Mean (Variable Frequency) : spsMeanVariableFrequencyLib/Mean (Variable Frequency)  Finit=Fnom  Fmin=f_min_pll  Vinit=0  Ts=Ts_Control
  Regulator : Subsystem  TreatAsAtomicUnit=on
  Sum : Sum  Inputs=1  SaturateOnIntegerOverflow=on
  Switch2 : Switch  Criteria=u2 > Threshold  InputSameDT=off
  dVref_abc : Outport  VectorParamsAs1DForOutWhenUnconnected=off
  Udc_0_mean : Outport  Port=2  VectorParamsAs1DForOutWhenUnconnected=off
  wires:
  First-Order Filter/1 -> Mean (Variable Frequency)/2
  Sum/1 -> First-Order Filter/1
  Freq/1 -> Mean (Variable Frequency)/1
  Vref_lim_abc/1 -> Regulator/1(V_ref_lim_abc)
  Iv_abc/1 -> Regulator/2(Iv_abc)
  Udc_pn/1 -> Sum/1
  Mean (Variable Frequency)/1 -> Gain4/1
  Gain4/1 -> Regulator/3(Udc_0_mean), Udc_0_mean/1
  Regulator/1(dV_ref_abc_dcvbc) -> Switch2/1
  Switch2/1 -> dVref_abc/1
  Constant8/1 -> Switch2/3
  activate_reg/1 -> Regulator/Enable, Switch2/2

== system HVDCVSCBased/VSC Controller Station 2/Discrete VSC Controller /Inner Current Loop ==
  note: Inner Current Loop
  U_dq : Inport
  Iv_dq : Inport  Port=2
  Udc_meas : Inport  Port=3
  Iref_dq : Inport  Port=4
  Freq : Inport  Port=5
  wt : Inport  Port=6
  AC_Current_Control : Subsystem
  Alpha-Beta-Zero to abc : spsAlphaBetaZerotoabcLib/Alpha-Beta-Zero to abc
  Constant1 : Constant  Value=0
  Max=10 Min=0 : Saturate  UpperLimit=10  LowerLimit=0
  Mean (Variable Frequency IC = 1.0 ) : spsMeanVariableFrequencyLib/Mean (Variable Frequency)  Finit=Fnom  Fmin=f_min_pll  Vinit=1.0  Ts=Ts_Control
  Mux1 : Mux  Inputs=[2 1]
  Reference_Voltage_Conditioning : Subsystem
  Reference_Voltage_Limitation : Subsystem
  Selector : Selector  InputPortWidth=3  IndexOptions=Index vector (dialog)  Indices=[ 1 2]  OutputSizes=1
  dq0 to Alpha-Beta-Zero : spsdq0toAlphaBetaZeroLib/dq0 to Alpha-Beta-Zero  Alignment=90 degrees behind phase A axis
  Vref_lim_abc : Outport  VectorParamsAs1DForOutWhenUnconnected=off
  Vref_lim_AB : Outport  Port=2  VectorParamsAs1DForOutWhenUnconnected=off
  wires:
  Udc_meas/1 -> Mean (Variable Frequency IC = 1.0 )/2
  Selector/1 -> Vref_lim_AB/1
  Reference_Voltage_Limitation/1(Vref_lim_dq) -> Mux1/1
  Alpha-Beta-Zero to abc/1 -> Vref_lim_abc/1
  Mux1/1 -> dq0 to Alpha-Beta-Zero/1
  Constant1/1 -> Mux1/2
  wt/1 -> dq0 to Alpha-Beta-Zero/2
  dq0 to Alpha-Beta-Zero/1 -> Selector/1, Alpha-Beta-Zero to abc/1
  Mean (Variable Frequency IC = 1.0 )/1 -> Max=10 Min=0/1
  Freq/1 -> Mean (Variable Frequency IC = 1.0 )/1, AC_Current_Control/4(Freq)
  Iref_dq/1 -> AC_Current_Control/2(Iref_dq)
  U_dq/1 -> AC_Current_Control/3(U_dq)
  Reference_Voltage_Conditioning/1(Vref_dq) -> Reference_Voltage_Limitation/1(Vref_dq)
  AC_Current_Control/1(Vref_dq_tmp) -> Reference_Voltage_Conditioning/1(Vref_dq_tmp)
  Max=10 Min=0/1 -> Reference_Voltage_Conditioning/2(Udc_meas_mean)
  Iv_dq/1 -> AC_Current_Control/1(Iv_dq)

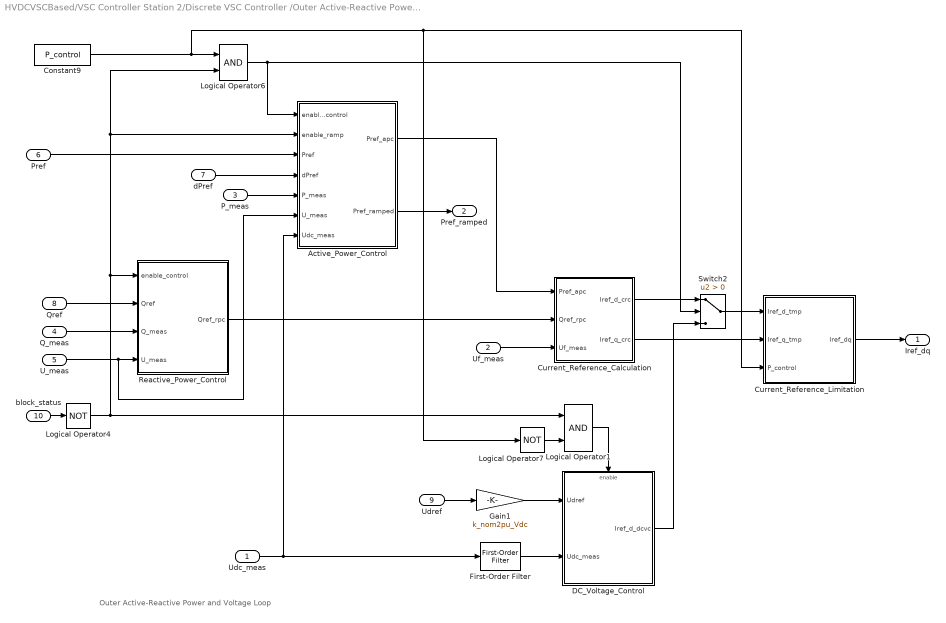
== system HVDCVSCBased/VSC Controller Station 2/Discrete VSC Controller /Outer Active-Reactive Power and Voltage Loop ==
  note: Outer Active-Reactive Power and Voltage Loop
  Udc_meas : Inport
  Uf_meas : Inport  Port=2
  P_meas : Inport  Port=3
  Q_meas : Inport  Port=4
  U_meas : Inport  Port=5
  Pref : Inport  Port=6
  dPref : Inport  Port=7
  Qref : Inport  Port=8
  Udref : Inport  Port=9
  block_status : Inport  Port=10
  Active_Power_Control : Subsystem
  Constant9 : Constant  Value=P_control
  Current_Reference_Calculation : Subsystem
  Current_Reference_Limitation : Subsystem
  DC_Voltage_Control : Subsystem
  First-Order Filter : spsFirstOrderFilterLib/First-Order Filter  FilterType=Lowpass  Tc=1/(2*pi*f0_Udc)  Ts=Ts_Control  Initialize=on  Vac_Init=[0, 0, 60]  Vdc_Init=k_nom2pu_Vdc  PlotResponse=off  FreqRange="[0,  200,  1]"
      settings: AttributesFormatString=Tc:%<Tc>\nIC:%<Vdc_Init>
  Gain1 : Gain  Gain=k_nom2pu_Vdc  SaturateOnIntegerOverflow=on  OutDataTypeStr=Inherit: Same as input  ParamDataTypeStr=Inherit: Same as input
      settings: AttributesFormatString=Gain:%<Gain>
  Logical Operator1 : Logic  AllPortsSameDT=off
  Logical Operator4 : Logic  Operator=NOT  AllPortsSameDT=off
  Logical Operator6 : Logic  AllPortsSameDT=off
  Logical Operator7 : Logic  Operator=NOT  AllPortsSameDT=off
  Reactive_Power_Control : Subsystem
  Switch2 : Switch  Criteria=u2 > Threshold  InputSameDT=off
  Iref_dq : Outport  VectorParamsAs1DForOutWhenUnconnected=off
  Pref_ramped : Outport  Port=2  VectorParamsAs1DForOutWhenUnconnected=off
  wires:
  First-Order Filter/1 -> DC_Voltage_Control/2(Udc_meas)
  Udref/1 -> Gain1/1
  Gain1/1 -> DC_Voltage_Control/1(Udref)
  Logical Operator1/1 -> DC_Voltage_Control/Enable
  Current_Reference_Limitation/1(Iref_dq) -> Iref_dq/1
  Switch2/1 -> Current_Reference_Limitation/1(Iref_d_tmp)
  Logical Operator4/1 -> Logical Operator1/1, Logical Operator6/2, Active_Power_Control/2(enable_ramp), Reactive_Power_Control/1(enable_control)
  Current_Reference_Calculation/1(Iref_d_crc) -> Switch2/1
  Q_meas/1 -> Reactive_Power_Control/3(Q_meas)
  P_meas/1 -> Active_Power_Control/5(P_meas)
  DC_Voltage_Control/1(Iref_d_dcvc) -> Switch2/3
  Udc_meas/1 -> Active_Power_Control/7(Udc_meas), First-Order Filter/1
  block_status/1 -> Logical Operator4/1
  Constant9/1 -> Logical Operator6/1, Current_Reference_Limitation/3(P_control), Logical Operator7/1
  Logical Operator6/1 -> Switch2/2, Active_Power_Control/1(enable_control)
  U_meas/1 -> Reactive_Power_Control/4(U_meas), Active_Power_Control/6(U_meas)
  Current_Reference_Calculation/2(Iref_q_crc) -> Current_Reference_Limitation/2(Iref_q_tmp)
  dPref/1 -> Active_Power_Control/4(dPref)
  Active_Power_Control/1(Pref_apc) -> Current_Reference_Calculation/1(Pref_apc)
  Reactive_Power_Control/1(Qref_rpc) -> Current_Reference_Calculation/2(Qref_rpc)
  Pref/1 -> Active_Power_Control/3(Pref)
  Uf_meas/1 -> Current_Reference_Calculation/3(Uf_meas)
  Qref/1 -> Reactive_Power_Control/2(Qref)
  Logical Operator7/1 -> Logical Operator1/2
  Active_Power_Control/2(Pref_ramped) -> Pref_ramped/1

== system HVDCVSCBased/VSC Controller Station 2/Discrete VSC Controller /PLL ==
  note: Discrete 3-phase PLL (Variation)
  U_AB : Inport
  Alpha-Beta-Zero to dq0 : spsAlphaBetaZerotodq0Lib/Alpha-Beta-Zero to dq0  Alignment=90 degrees behind phase A axis
  Constant1 : Constant  Value=0
  Constant4 : Constant  Value=2*pi
  Discrete PI Controller : Subsystem  DialogController=POWERSYS.PowerSysDialog  mask(Discrete PI Controller){Kp=Kp, Ki=Ki, Par_Limits=2*pi*Finit*[1.25 0.75], Init=2*pi*Finit, Ts=Ts}
      mask prompts: Kp "Proportional gain (Kp):"; Ki "Integral gain (Ki):"; Par_Limits "Output limits: [ Upper   Lower ]"; Init "Output initial value:"; Ts "Sample time:"
      mask help: This block implements a discrete PI controller.
      mask init:
      | UpperLimit=Par_Limits(1);
      | LowerLimit=Par_Limits(2);
      | power_initmask();
      mask Help: This block is part of a subset of blocks in the Extras library that does not have documentation associated with it, other than the block mask description.
      mask Display: disp('PI');
  Discrete Rate Limiter : Subsystem  DialogController=POWERSYS.PowerSysDialog  mask(Discrete Rate Limiter){R=12, F=-12, Vinit=Finit, Ts=Ts}
      mask prompts: R "Rising slew rate:"; F "Falling slew rate:"; Vinit "Initial input:"; Ts "Sample time:"
      mask help: DISCRETE BLOCK : Limit rising and falling rates of signal
      mask init:
      | UpperLimit=R*Ts;
      | LowerLimit=F*Ts;
      | power_initmask();
      mask Help: This block is part of a subset of blocks in the Extras library that does not have documentation associated with it, other than the block mask description.
      mask Display: disp('Discrete\nRate\nLimiter')
  Discrete-Time Integrator : DiscreteIntegrator  InitialCondition=Phase_Init*pi/180  SampleTime=Ts  ICPrevOutput=DiscIntNeverNeededParam  ICPrevScaledInput=DiscIntNeverNeededParam
  Gain10 : Gain  Gain=1/2/pi  SaturateOnIntegerOverflow=on  OutDataTypeStr=Inherit: Same as input  ParamDataTypeStr=Inherit: Same as input
  Math Function : Math  Operator=mod  SignedPower=on
  Mean (Variable Frequency) : spsMeanVariableFrequencyLib/Mean (Variable Frequency)  Finit=Finit  Fmin=Fmin  Vinit=0  Ts=Ts
  Mux1 : Mux  Inputs=[2 1]
  Second-Order Filter : spsSecondOrderFilterLib/Second-Order Filter  FilterType=Lowpass  Fo=25  Zeta=0.707  Ts=Ts  Initialize=on  Vac_Init=[0 0 Finit]  Vdc_Init=Finit  PlotResponse=off  FreqRange=[0, 500, 1]
  Selector : Selector  InputPortWidth=3  IndexOptions=Index vector (dialog)  Indices=2  OutputSizes=1
  Unit Delay : UnitDelay  InitialCondition=Finit  SampleTime=Ts  HasFrameUpgradeWarning=on
  Freq : Outport  VectorParamsAs1DForOutWhenUnconnected=off
  wt : Outport  Port=2  VectorParamsAs1DForOutWhenUnconnected=off
  wires:
  Constant1/1 -> Mux1/2
  Mux1/1 -> Alpha-Beta-Zero to dq0/1
  U_AB/1 -> Mux1/1
  Mean (Variable Frequency)/1 -> Discrete PI Controller/1(Error)
  Alpha-Beta-Zero to dq0/1 -> Selector/1
  Constant4/1 -> Math Function/2
  Discrete-Time Integrator/1 -> Math Function/1
  Math Function/1 -> wt/1, Alpha-Beta-Zero to dq0/2
  Discrete PI Controller/1(Out) -> Discrete-Time Integrator/1, Gain10/1  "W"
  Gain10/1 -> Discrete Rate Limiter/1(In)
  Discrete Rate Limiter/1(Out) -> Second-Order Filter/1
  Unit Delay/1 -> Freq/1, Mean (Variable Frequency)/1
  Second-Order Filter/1 -> Unit Delay/1
  Selector/1 -> Mean (Variable Frequency)/2  "Vq"

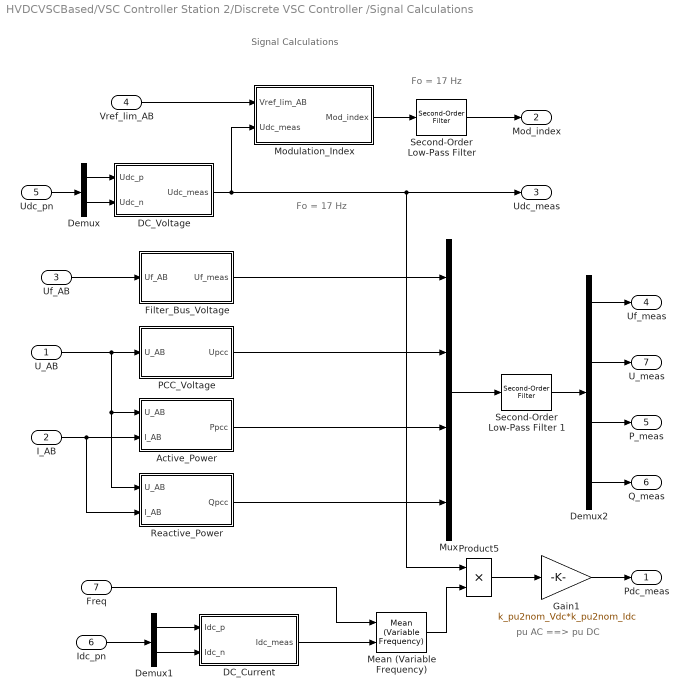
== system HVDCVSCBased/VSC Controller Station 2/Discrete VSC Controller /Signal Calculations ==
  note: Fo = 17 Hz
  note: Fo = 17 Hz
  note: Signal Calculations
  note: pu AC ==> pu DC
  U_AB : Inport
  I_AB : Inport  Port=2
  Uf_AB : Inport  Port=3
  Vref_lim_AB : Inport  Port=4
  Udc_pn : Inport  Port=5
  Idc_pn : Inport  Port=6
  Freq : Inport  Port=7
  Active_Power : Subsystem
  DC_Current : Subsystem
  DC_Voltage : Subsystem
  Demux : Demux  Outputs=2
      settings: DisplayOption=none
  Demux1 : Demux  Outputs=2
      settings: DisplayOption=none
  Demux2 : Demux
  Filter_Bus_Voltage : Subsystem
  Gain1 : Gain  Gain=k_pu2nom_Vdc*k_pu2nom_Idc  SaturateOnIntegerOverflow=on  OutDataTypeStr=Inherit: Same as input  ParamDataTypeStr=Inherit: Same as input
  "Mean (Variable Frequency) " : spsMeanVariableFrequencyLib/Mean (Variable Frequency)  Finit=Fnom  Fmin=f_min_pll  Vinit=0  Ts=Ts_Control
  Modulation_Index : Subsystem
  Mux : Mux
  PCC_Voltage : Subsystem
  Product5 : Product  SaturateOnIntegerOverflow=on  OutDataTypeStr=Inherit: Same as first input
  Reactive_Power : Subsystem
  "Second-Order Low-Pass Filter " : spsSecondOrderFilterLib/Second-Order Filter  FilterType=Lowpass  Fo=f0_sc  Zeta=zeta_sc  Ts=Ts_Control  Initialize=off  Vac_Init="[0,  0,  60]"  Vdc_Init=0  PlotResponse=off  FreqRange=[0, 500, 1]
      settings: AttributesFormatString=f0=%<Fo>
  Second-Order Low-Pass Filter 1 : spsSecondOrderFilterLib/Second-Order Filter  FilterType=Lowpass  Fo=f0_sc  Zeta=zeta_sc  Ts=Ts_Control  Initialize=off  Vac_Init="[0,  0,  60]"  Vdc_Init=0  PlotResponse=off  FreqRange=[0, 500, 1]
      settings: AttributesFormatString=f0=%<Fo>
  Pdc_meas : Outport  VectorParamsAs1DForOutWhenUnconnected=off
  Mod_index : Outport  Port=2  VectorParamsAs1DForOutWhenUnconnected=off
  Udc_meas : Outport  Port=3  VectorParamsAs1DForOutWhenUnconnected=off
  Uf_meas : Outport  Port=4  VectorParamsAs1DForOutWhenUnconnected=off
  P_meas : Outport  Port=5  VectorParamsAs1DForOutWhenUnconnected=off
  Q_meas : Outport  Port=6  VectorParamsAs1DForOutWhenUnconnected=off
  U_meas : Outport  Port=7  VectorParamsAs1DForOutWhenUnconnected=off
  wires:
  Demux2/4 -> Q_meas/1
  Demux2/3 -> P_meas/1
  Demux2/2 -> U_meas/1
  Demux2/1 -> Uf_meas/1
  Reactive_Power/1(Qpcc) -> Mux/4
  Active_Power/1(Ppcc) -> Mux/3
  PCC_Voltage/1(Upcc) -> Mux/2
  Filter_Bus_Voltage/1(Uf_meas) -> Mux/1
  "Second-Order Low-Pass Filter "/1 -> Mod_index/1
  Modulation_Index/1(Mod_index) -> "Second-Order Low-Pass Filter "/1
  Second-Order Low-Pass Filter 1/1 -> Demux2/1
  Mux/1 -> Second-Order Low-Pass Filter 1/1
  Gain1/1 -> Pdc_meas/1
  Freq/1 -> "Mean (Variable Frequency) "/1
  Product5/1 -> Gain1/1
  "Mean (Variable Frequency) "/1 -> Product5/2
  Demux/2 -> DC_Voltage/2(Udc_n)
  Uf_AB/1 -> Filter_Bus_Voltage/1(Uf_AB)
  U_AB/1 -> PCC_Voltage/1(U_AB), Active_Power/1(U_AB), Reactive_Power/1(U_AB)
  I_AB/1 -> Active_Power/2(I_AB), Reactive_Power/2(I_AB)
  DC_Voltage/1(Udc_meas) -> Product5/1, Udc_meas/1, Modulation_Index/2(Udc_meas)
  DC_Current/1(Idc_meas) -> "Mean (Variable Frequency) "/2
  Udc_pn/1 -> Demux/1
  Demux/1 -> DC_Voltage/1(Udc_p)
  Demux1/1 -> DC_Current/1(Idc_p)
  Demux1/2 -> DC_Current/2(Idc_n)
  Idc_pn/1 -> Demux1/1
  Vref_lim_AB/1 -> Modulation_Index/1(Vref_lim_AB)

== system HVDCVSCBased/VSC Controller Station 2/Discrete VSC Controller /dq Transformations ==
  note: dq Transformations
  U_AB : Inport
  Iv_AB : Inport  Port=2
  wt : Inport  Port=3
  Alpha-Beta-Zero to dq0 : spsAlphaBetaZerotodq0Lib/Alpha-Beta-Zero to dq0  Alignment=90 degrees behind phase A axis
  "Alpha-Beta-Zero to dq0 " : spsAlphaBetaZerotodq0Lib/Alpha-Beta-Zero to dq0  Alignment=90 degrees behind phase A axis
  Constant1 : Constant  Value=0
  Mux1 : Mux  Inputs=[2 1]
  Mux4 : Mux  Inputs=[2 1]
  Selector : Selector  InputPortWidth=3  IndexOptions=Index vector (dialog)  Indices=[1 2]  OutputSizes=1
  Selector3 : Selector  InputPortWidth=3  IndexOptions=Index vector (dialog)  Indices=[1 2]  OutputSizes=1
  U_dq : Outport  VectorParamsAs1DForOutWhenUnconnected=off
  Iv_dq : Outport  Port=2  VectorParamsAs1DForOutWhenUnconnected=off
  wires:
  wt/1 -> Alpha-Beta-Zero to dq0/2, "Alpha-Beta-Zero to dq0 "/2
  Constant1/1 -> Mux4/2, Mux1/2
  Mux4/1 -> "Alpha-Beta-Zero to dq0 "/1
  Iv_AB/1 -> Mux4/1
  Mux1/1 -> Alpha-Beta-Zero to dq0/1
  U_AB/1 -> Mux1/1
  "Alpha-Beta-Zero to dq0 "/1 -> Selector3/1
  Alpha-Beta-Zero to dq0/1 -> Selector/1
  Selector/1 -> U_dq/1
  Selector3/1 -> Iv_dq/1

== system HVDCVSCBased/VSC Controller Station 1/Discrete VSC Controller /Clark Transformations/CLARK  with Rotating reference ==
  note: Rotation of pi/6
  note: Rotation of - pi/6
  note: Reference rotation:
      | Type [0,1,2]          Rotation (rad)
      | 0                            0
      | 1                            - pi/6
      | 2                              pi/6
  note: CLARK transformations
  abc : Inport
  Type : Inport  Port=2
  CLARK : Subsystem  TreatAsAtomicUnit=on
  CLARK_lag : Subsystem  TreatAsAtomicUnit=on
  CLARK_lead : Subsystem  TreatAsAtomicUnit=on
  Constant : Constant  Value=2
  Constant1 : Constant  Value=0
  Constant2 : Constant
  Relational Operator1 : RelationalOperator  Operator===
  Relational Operator2 : RelationalOperator  Operator===
  Relational Operator3 : RelationalOperator  Operator===
  Sum : Sum  Inputs=+++  SaturateOnIntegerOverflow=on
  AB0 : Outport  VectorParamsAs1DForOutWhenUnconnected=off
  wires:
  Constant2/1 -> Relational Operator3/2
  Relational Operator2/1 -> CLARK/Enable
  Constant1/1 -> Relational Operator2/2
  CLARK/1(AB0) -> Sum/3
  Sum/1 -> AB0/1
  CLARK_lag/1(AB0) -> Sum/2
  CLARK_lead/1(AB0) -> Sum/1
  abc/1 -> CLARK/1(abc), CLARK_lag/1(abc), CLARK_lead/1(abc)
  Relational Operator1/1 -> CLARK_lead/Enable
  Relational Operator3/1 -> CLARK_lag/Enable
  Type/1 -> Relational Operator3/1, Relational Operator2/1, Relational Operator1/1
  Constant/1 -> Relational Operator1/2

== system HVDCVSCBased/VSC Controller Station 1/Discrete VSC Controller /Clark Transformations/CLARK  with Rotating reference1 ==
  note: Rotation of pi/6
  note: Rotation of - pi/6
  note: Reference rotation:
      | Type [0,1,2]          Rotation (rad)
      | 0                            0
      | 1                            - pi/6
      | 2                              pi/6
  note: CLARK transformations
  abc : Inport
  Type : Inport  Port=2
  CLARK : Subsystem  TreatAsAtomicUnit=on
  CLARK_lag : Subsystem  TreatAsAtomicUnit=on
  CLARK_lead : Subsystem  TreatAsAtomicUnit=on
  Constant : Constant  Value=2
  Constant1 : Constant  Value=0
  Constant2 : Constant
  Relational Operator1 : RelationalOperator  Operator===
  Relational Operator2 : RelationalOperator  Operator===
  Relational Operator3 : RelationalOperator  Operator===
  Sum : Sum  Inputs=+++  SaturateOnIntegerOverflow=on
  AB0 : Outport  VectorParamsAs1DForOutWhenUnconnected=off
  wires:
  Constant2/1 -> Relational Operator3/2
  Relational Operator2/1 -> CLARK/Enable
  Constant1/1 -> Relational Operator2/2
  CLARK/1(AB0) -> Sum/3
  Sum/1 -> AB0/1
  CLARK_lag/1(AB0) -> Sum/2
  CLARK_lead/1(AB0) -> Sum/1
  abc/1 -> CLARK/1(abc), CLARK_lag/1(abc), CLARK_lead/1(abc)
  Relational Operator1/1 -> CLARK_lead/Enable
  Relational Operator3/1 -> CLARK_lag/Enable
  Type/1 -> Relational Operator3/1, Relational Operator2/1, Relational Operator1/1
  Constant/1 -> Relational Operator1/2
